simulink model "Lab_8"  (R2014a)
settings: Solver=ode23t  StartTime=0.0  StopTime=20  RelTol=1e-3
settings Model: Creator=cloughj  LastModifiedBy=cloughj
settings SolverCC: ZeroCrossAlgorithm=Adaptive

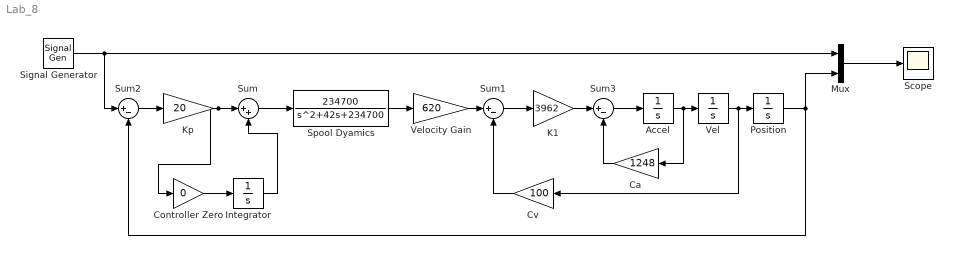
== system Lab_8 ==
  Accel : Integrator
  Ca : Gain  Gain=1248
  Controller Zero : Gain  Gain=0
  Cv : Gain  Gain=100
  Integrator : Integrator
  K1 : Gain  Gain=3962
  Kp : Gain  Gain=20
  Mux : Mux  Inputs=2
  Position : Integrator
  Scope : Scope
  Signal Generator : SignalGenerator  WaveForm=square  Frequency=0.1
  Spool Dyamics : TransferFcn  Numerator=[234700]  Denominator=[1 42 234700]
  Sum : Sum  Inputs=|++
  Sum1 : Sum  Inputs=|+-
  Sum2 : Sum  Inputs=|+-
  Sum3 : Sum  Inputs=|+-
  Vel : Integrator
  Velocity Gain : Gain  Gain=620
  wires:
  Mux/1 -> Scope/1
  Signal Generator/1 -> Sum2/1, Mux/1
  Velocity Gain/1 -> Sum1/1
  Cv/1 -> Sum1/2
  Position/1 -> Sum2/2, Mux/2
  Sum2/1 -> Kp/1
  Kp/1 -> Controller Zero/1, Sum/1
  Sum/1 -> Spool Dyamics/1
  Controller Zero/1 -> Integrator/1
  Integrator/1 -> Sum/2
  Spool Dyamics/1 -> Velocity Gain/1
  Sum1/1 -> K1/1
  K1/1 -> Sum3/1
  Sum3/1 -> Accel/1
  Accel/1 -> Ca/1, Vel/1
  Vel/1 -> Cv/1, Position/1
  Ca/1 -> Sum3/2
